simulink model "fft_wideband_real"  (R2012b)
settings: Solver=ode45  StartTime=0.0  StopTime=19999  RelTol=1e-3
undefined symbols (not defined in the file): fft_wideband_real_shift_schedule_user_data_out
libraries: xbsIndex_r4 x8703, xbsReplacements_r4 x36, xps_library x24, dspsigops x16, simulink_xsg_bridge x1
(part 2 of 51)

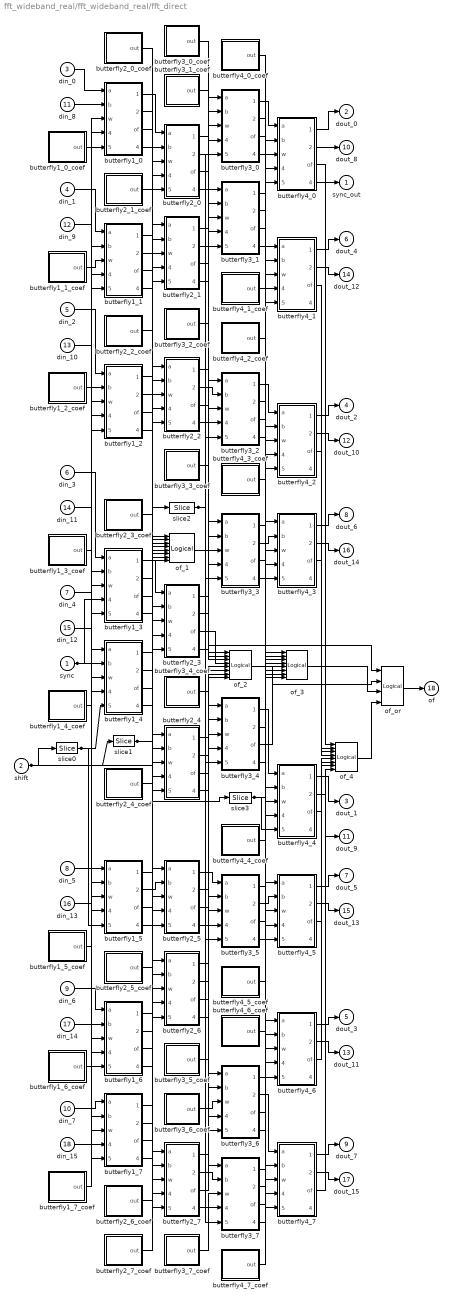
== system fft_wideband_real/fft_wideband_real/fft_direct ==
  sync : Inport
  shift : Inport  Port=2
  din_0 : Inport  Port=3
  din_1 : Inport  Port=4
  din_2 : Inport  Port=5
  din_3 : Inport  Port=6
  din_4 : Inport  Port=7
  din_5 : Inport  Port=8
  din_6 : Inport  Port=9
  din_7 : Inport  Port=10
  din_8 : Inport  Port=11
  din_9 : Inport  Port=12
  din_10 : Inport  Port=13
  din_11 : Inport  Port=14
  din_12 : Inport  Port=15
  din_13 : Inport  Port=16
  din_14 : Inport  Port=17
  din_15 : Inport  Port=18
  butterfly1_0 : Subsystem
      settings: AttributesFormatString=|
      | twiddle_pass_through
      | coeffs in slices
      | Bit growth:0
  butterfly1_0_coef : Subsystem
  butterfly1_1 : Subsystem
      settings: AttributesFormatString=|
      | twiddle_pass_through
      | coeffs in slices
      | Bit growth:0
  butterfly1_1_coef : Subsystem
  butterfly1_2 : Subsystem
      settings: AttributesFormatString=|
      | twiddle_pass_through
      | coeffs in slices
      | Bit growth:0
  butterfly1_2_coef : Subsystem
  butterfly1_3 : Subsystem
      settings: AttributesFormatString=|
      | twiddle_pass_through
      | coeffs in slices
      | Bit growth:0
  butterfly1_3_coef : Subsystem
  butterfly1_4 : Subsystem
      settings: AttributesFormatString=|
      | twiddle_pass_through
      | coeffs in slices
      | Bit growth:0
  butterfly1_4_coef : Subsystem
  butterfly1_5 : Subsystem
      settings: AttributesFormatString=|
      | twiddle_pass_through
      | coeffs in slices
      | Bit growth:0
  butterfly1_5_coef : Subsystem
  butterfly1_6 : Subsystem
      settings: AttributesFormatString=|
      | twiddle_pass_through
      | coeffs in slices
      | Bit growth:0
  butterfly1_6_coef : Subsystem
  butterfly1_7 : Subsystem
      settings: AttributesFormatString=|
      | twiddle_pass_through
      | coeffs in slices
      | Bit growth:0
  butterfly1_7_coef : Subsystem
  butterfly2_0 : Subsystem
      settings: AttributesFormatString=|
      | twiddle_pass_through
      | coeffs in slices
      | Bit growth:0
  butterfly2_0_coef : Subsystem
  butterfly2_1 : Subsystem
      settings: AttributesFormatString=|
      | twiddle_pass_through
      | coeffs in slices
      | Bit growth:0
  butterfly2_1_coef : Subsystem
  butterfly2_2 : Subsystem
      settings: AttributesFormatString=|
      | twiddle_pass_through
      | coeffs in slices
      | Bit growth:0
  butterfly2_2_coef : Subsystem
  butterfly2_3 : Subsystem
      settings: AttributesFormatString=|
      | twiddle_pass_through
      | coeffs in slices
      | Bit growth:0
  butterfly2_3_coef : Subsystem
  butterfly2_4 : Subsystem
      settings: AttributesFormatString=|
      | twiddle_coeff_1
      | coeffs in slices
      | Bit growth:0
  butterfly2_4_coef : Subsystem
  butterfly2_5 : Subsystem
      settings: AttributesFormatString=|
      | twiddle_coeff_1
      | coeffs in slices
      | Bit growth:0
  butterfly2_5_coef : Subsystem
  butterfly2_6 : Subsystem
      settings: AttributesFormatString=|
      | twiddle_coeff_1
      | coeffs in slices
      | Bit growth:0
  butterfly2_6_coef : Subsystem
  butterfly2_7 : Subsystem
      settings: AttributesFormatString=|
      | twiddle_coeff_1
      | coeffs in slices
      | Bit growth:0
  butterfly2_7_coef : Subsystem
  butterfly3_0 : Subsystem
      settings: AttributesFormatString=|
      | twiddle_general_4mult
      | coeffs in slices
      | Bit growth:0
  butterfly3_0_coef : Subsystem
  butterfly3_1 : Subsystem
      settings: AttributesFormatString=|
      | twiddle_general_4mult
      | coeffs in slices
      | Bit growth:0
  butterfly3_1_coef : Subsystem
  butterfly3_2 : Subsystem
      settings: AttributesFormatString=|
      | twiddle_general_4mult
      | coeffs in slices
      | Bit growth:0
  butterfly3_2_coef : Subsystem
  butterfly3_3 : Subsystem
      settings: AttributesFormatString=|
      | twiddle_general_4mult
      | coeffs in slices
      | Bit growth:0
  butterfly3_3_coef : Subsystem
  butterfly3_4 : Subsystem
      settings: AttributesFormatString=|
      | twiddle_general_4mult
      | coeffs in slices
      | Bit growth:0
  butterfly3_4_coef : Subsystem
  butterfly3_5 : Subsystem
      settings: AttributesFormatString=|
      | twiddle_general_4mult
      | coeffs in slices
      | Bit growth:0
  butterfly3_5_coef : Subsystem
  butterfly3_6 : Subsystem
      settings: AttributesFormatString=|
      | twiddle_general_4mult
      | coeffs in slices
      | Bit growth:0
  butterfly3_6_coef : Subsystem
  butterfly3_7 : Subsystem
      settings: AttributesFormatString=|
      | twiddle_general_4mult
      | coeffs in slices
      | Bit growth:0
  butterfly3_7_coef : Subsystem
  butterfly4_0 : Subsystem
      settings: AttributesFormatString=|
      | twiddle_general_4mult
      | coeffs in slices
      | Bit growth:0
  butterfly4_0_coef : Subsystem
  butterfly4_1 : Subsystem
      settings: AttributesFormatString=|
      | twiddle_general_4mult
      | coeffs in slices
      | Bit growth:0
  butterfly4_1_coef : Subsystem
  butterfly4_2 : Subsystem
      settings: AttributesFormatString=|
      | twiddle_general_4mult
      | coeffs in slices
      | Bit growth:0
  butterfly4_2_coef : Subsystem
  butterfly4_3 : Subsystem
      settings: AttributesFormatString=|
      | twiddle_general_4mult
      | coeffs in slices
      | Bit growth:0
  butterfly4_3_coef : Subsystem
  butterfly4_4 : Subsystem
      settings: AttributesFormatString=|
      | twiddle_general_4mult
      | coeffs in slices
      | Bit growth:0
  butterfly4_4_coef : Subsystem
  butterfly4_5 : Subsystem
      settings: AttributesFormatString=|
      | twiddle_general_4mult
      | coeffs in slices
      | Bit growth:0
  butterfly4_5_coef : Subsystem
  butterfly4_6 : Subsystem
      settings: AttributesFormatString=|
      | twiddle_general_4mult
      | coeffs in slices
      | Bit growth:0
  butterfly4_6_coef : Subsystem
  butterfly4_7 : Subsystem
      settings: AttributesFormatString=|
      | twiddle_general_4mult
      | coeffs in slices
      | Bit growth:0
  butterfly4_7_coef : Subsystem
  of_{1..4} (4 alike) : xbsIndex_r4/Logical  logical_function=OR  inputs=8  en=off  latency=1  precision=Full  arith_type=Unsigned  n_bits=16  bin_pt=0  align_bp=on  dbl_ovrd=off  block_type=logical
  of_or : xbsIndex_r4/Logical  logical_function=OR  inputs=4  en=off  latency=0  precision=Full  arith_type=Unsigned  n_bits=16  bin_pt=0  align_bp=on  dbl_ovrd=off  block_type=logical
  slice0 : xbsIndex_r4/Slice  nbits=1  boolean_output=on  mode=Lower Bit Location + Width  bit1=0  base1=MSB of Input  bit0=0  base0=LSB of Input  dbl_ovrd=off  block_type=slice
  slice1 : xbsIndex_r4/Slice  nbits=1  boolean_output=on  mode=Lower Bit Location + Width  bit1=0  base1=MSB of Input  bit0=1  base0=LSB of Input  dbl_ovrd=off  block_type=slice
  slice2 : xbsIndex_r4/Slice  nbits=1  boolean_output=on  mode=Lower Bit Location + Width  bit1=0  base1=MSB of Input  bit0=2  base0=LSB of Input  dbl_ovrd=off  block_type=slice
  slice3 : xbsIndex_r4/Slice  nbits=1  boolean_output=on  mode=Lower Bit Location + Width  bit1=0  base1=MSB of Input  bit0=3  base0=LSB of Input  dbl_ovrd=off  block_type=slice
  sync_out : Outport
  dout_0 : Outport  Port=2
  dout_1 : Outport  Port=3
  dout_2 : Outport  Port=4
  dout_3 : Outport  Port=5
  dout_4 : Outport  Port=6
  dout_5 : Outport  Port=7
  dout_6 : Outport  Port=8
  dout_7 : Outport  Port=9
  dout_8 : Outport  Port=10
  dout_9 : Outport  Port=11
  dout_10 : Outport  Port=12
  dout_11 : Outport  Port=13
  dout_12 : Outport  Port=14
  dout_13 : Outport  Port=15
  dout_14 : Outport  Port=16
  dout_15 : Outport  Port=17
  of : Outport  Port=18
  wires:
  din_0/1 -> butterfly1_0/1(a)
  din_8/1 -> butterfly1_0/2(b)
  butterfly1_0_coef/1(out) -> butterfly1_0/3(w)
  din_1/1 -> butterfly1_1/1(a)
  din_9/1 -> butterfly1_1/2(b)
  butterfly1_1_coef/1(out) -> butterfly1_1/3(w)
  din_2/1 -> butterfly1_2/1(a)
  din_10/1 -> butterfly1_2/2(b)
  butterfly1_2_coef/1(out) -> butterfly1_2/3(w)
  din_3/1 -> butterfly1_3/1(a)
  din_11/1 -> butterfly1_3/2(b)
  butterfly1_3_coef/1(out) -> butterfly1_3/3(w)
  din_4/1 -> butterfly1_4/1(a)
  din_12/1 -> butterfly1_4/2(b)
  butterfly1_4_coef/1(out) -> butterfly1_4/3(w)
  din_5/1 -> butterfly1_5/1(a)
  din_13/1 -> butterfly1_5/2(b)
  butterfly1_5_coef/1(out) -> butterfly1_5/3(w)
  din_6/1 -> butterfly1_6/1(a)
  din_14/1 -> butterfly1_6/2(b)
  butterfly1_6_coef/1(out) -> butterfly1_6/3(w)
  din_7/1 -> butterfly1_7/1(a)
  din_15/1 -> butterfly1_7/2(b)
  butterfly1_7_coef/1(out) -> butterfly1_7/3(w)
  butterfly1_0/3(of) -> of_1/1
  butterfly1_1/3(of) -> of_1/2
  butterfly1_2/3(of) -> of_1/3
  butterfly1_3/3(of) -> of_1/4
  butterfly1_4/3(of) -> of_1/5
  butterfly1_5/3(of) -> of_1/6
  butterfly1_6/3(of) -> of_1/7
  butterfly1_7/3(of) -> of_1/8
  butterfly1_0/1(a+bw) -> butterfly2_0/1(a)
  butterfly1_4/1(a+bw) -> butterfly2_0/2(b)
  butterfly2_0_coef/1(out) -> butterfly2_0/3(w)
  butterfly1_0/4(sync_out) -> butterfly2_0/4(sync)
  butterfly1_1/1(a+bw) -> butterfly2_1/1(a)
  butterfly1_5/1(a+bw) -> butterfly2_1/2(b)
  butterfly2_1_coef/1(out) -> butterfly2_1/3(w)
  butterfly1_1/4(sync_out) -> butterfly2_1/4(sync)
  butterfly1_2/1(a+bw) -> butterfly2_2/1(a)
  butterfly1_6/1(a+bw) -> butterfly2_2/2(b)
  butterfly2_2_coef/1(out) -> butterfly2_2/3(w)
  butterfly1_2/4(sync_out) -> butterfly2_2/4(sync)
  butterfly1_3/1(a+bw) -> butterfly2_3/1(a)
  butterfly1_7/1(a+bw) -> butterfly2_3/2(b)
  butterfly2_3_coef/1(out) -> butterfly2_3/3(w)
  butterfly1_3/4(sync_out) -> butterfly2_3/4(sync)
  butterfly1_0/2(a-bw) -> butterfly2_4/1(a)
  butterfly1_4/2(a-bw) -> butterfly2_4/2(b)
  butterfly2_4_coef/1(out) -> butterfly2_4/3(w)
  butterfly1_4/4(sync_out) -> butterfly2_4/4(sync)
  butterfly1_1/2(a-bw) -> butterfly2_5/1(a)
  butterfly1_5/2(a-bw) -> butterfly2_5/2(b)
  butterfly2_5_coef/1(out) -> butterfly2_5/3(w)
  butterfly1_5/4(sync_out) -> butterfly2_5/4(sync)
  butterfly1_2/2(a-bw) -> butterfly2_6/1(a)
  butterfly1_6/2(a-bw) -> butterfly2_6/2(b)
  butterfly2_6_coef/1(out) -> butterfly2_6/3(w)
  butterfly1_6/4(sync_out) -> butterfly2_6/4(sync)
  butterfly1_3/2(a-bw) -> butterfly2_7/1(a)
  butterfly1_7/2(a-bw) -> butterfly2_7/2(b)
  butterfly2_7_coef/1(out) -> butterfly2_7/3(w)
  butterfly1_7/4(sync_out) -> butterfly2_7/4(sync)
  butterfly2_0/3(of) -> of_2/1
  butterfly2_1/3(of) -> of_2/2
  butterfly2_2/3(of) -> of_2/3
  butterfly2_3/3(of) -> of_2/4
  butterfly2_4/3(of) -> of_2/5
  butterfly2_5/3(of) -> of_2/6
  butterfly2_6/3(of) -> of_2/7
  butterfly2_7/3(of) -> of_2/8
  butterfly2_0/1(a+bw) -> butterfly3_0/1(a)
  butterfly2_2/1(a+bw) -> butterfly3_0/2(b)
  butterfly3_0_coef/1(out) -> butterfly3_0/3(w)
  butterfly2_0/4(sync_out) -> butterfly3_0/4(sync)
  butterfly2_1/1(a+bw) -> butterfly3_1/1(a)
  butterfly2_3/1(a+bw) -> butterfly3_1/2(b)
  butterfly3_1_coef/1(out) -> butterfly3_1/3(w)
  butterfly2_1/4(sync_out) -> butterfly3_1/4(sync)
  butterfly2_0/2(a-bw) -> butterfly3_2/1(a)
  butterfly2_2/2(a-bw) -> butterfly3_2/2(b)
  butterfly3_2_coef/1(out) -> butterfly3_2/3(w)
  butterfly2_2/4(sync_out) -> butterfly3_2/4(sync)
  butterfly2_1/2(a-bw) -> butterfly3_3/1(a)
  butterfly2_3/2(a-bw) -> butterfly3_3/2(b)
  butterfly3_3_coef/1(out) -> butterfly3_3/3(w)
  butterfly2_3/4(sync_out) -> butterfly3_3/4(sync)
  butterfly2_4/1(a+bw) -> butterfly3_4/1(a)
  butterfly2_6/1(a+bw) -> butterfly3_4/2(b)
  butterfly3_4_coef/1(out) -> butterfly3_4/3(w)
  butterfly2_4/4(sync_out) -> butterfly3_4/4(sync)
  butterfly2_5/1(a+bw) -> butterfly3_5/1(a)
  butterfly2_7/1(a+bw) -> butterfly3_5/2(b)
  butterfly3_5_coef/1(out) -> butterfly3_5/3(w)
  butterfly2_5/4(sync_out) -> butterfly3_5/4(sync)
  butterfly2_4/2(a-bw) -> butterfly3_6/1(a)
  butterfly2_6/2(a-bw) -> butterfly3_6/2(b)
  butterfly3_6_coef/1(out) -> butterfly3_6/3(w)
  butterfly2_6/4(sync_out) -> butterfly3_6/4(sync)
  butterfly2_5/2(a-bw) -> butterfly3_7/1(a)
  butterfly2_7/2(a-bw) -> butterfly3_7/2(b)
  butterfly3_7_coef/1(out) -> butterfly3_7/3(w)
  butterfly2_7/4(sync_out) -> butterfly3_7/4(sync)
  butterfly3_0/3(of) -> of_3/1
  butterfly3_1/3(of) -> of_3/2
  butterfly3_2/3(of) -> of_3/3
  butterfly3_3/3(of) -> of_3/4
  butterfly3_4/3(of) -> of_3/5
  butterfly3_5/3(of) -> of_3/6
  butterfly3_6/3(of) -> of_3/7
  butterfly3_7/3(of) -> of_3/8
  butterfly3_0/1(a+bw) -> butterfly4_0/1(a)
  butterfly3_1/1(a+bw) -> butterfly4_0/2(b)
  butterfly4_0_coef/1(out) -> butterfly4_0/3(w)
  butterfly3_0/4(sync_out) -> butterfly4_0/4(sync)
  butterfly4_0/4(sync_out) -> sync_out/1
  butterfly3_0/2(a-bw) -> butterfly4_1/1(a)
  butterfly3_1/2(a-bw) -> butterfly4_1/2(b)
  butterfly4_1_coef/1(out) -> butterfly4_1/3(w)
  butterfly3_1/4(sync_out) -> butterfly4_1/4(sync)
  butterfly3_2/1(a+bw) -> butterfly4_2/1(a)
  butterfly3_3/1(a+bw) -> butterfly4_2/2(b)
  butterfly4_2_coef/1(out) -> butterfly4_2/3(w)
  butterfly3_2/4(sync_out) -> butterfly4_2/4(sync)
  butterfly3_2/2(a-bw) -> butterfly4_3/1(a)
  butterfly3_3/2(a-bw) -> butterfly4_3/2(b)
  butterfly4_3_coef/1(out) -> butterfly4_3/3(w)
  butterfly3_3/4(sync_out) -> butterfly4_3/4(sync)
  butterfly3_4/1(a+bw) -> butterfly4_4/1(a)
  butterfly3_5/1(a+bw) -> butterfly4_4/2(b)
  butterfly4_4_coef/1(out) -> butterfly4_4/3(w)
  butterfly3_4/4(sync_out) -> butterfly4_4/4(sync)
  butterfly3_4/2(a-bw) -> butterfly4_5/1(a)
  butterfly3_5/2(a-bw) -> butterfly4_5/2(b)
  butterfly4_5_coef/1(out) -> butterfly4_5/3(w)
  butterfly3_5/4(sync_out) -> butterfly4_5/4(sync)
  butterfly3_6/1(a+bw) -> butterfly4_6/1(a)
  butterfly3_7/1(a+bw) -> butterfly4_6/2(b)
  butterfly4_6_coef/1(out) -> butterfly4_6/3(w)
  butterfly3_6/4(sync_out) -> butterfly4_6/4(sync)
  butterfly3_6/2(a-bw) -> butterfly4_7/1(a)
  butterfly3_7/2(a-bw) -> butterfly4_7/2(b)
  butterfly4_7_coef/1(out) -> butterfly4_7/3(w)
  butterfly3_7/4(sync_out) -> butterfly4_7/4(sync)
  butterfly4_0/3(of) -> of_4/1
  butterfly4_1/3(of) -> of_4/2
  butterfly4_2/3(of) -> of_4/3
  butterfly4_3/3(of) -> of_4/4
  butterfly4_4/3(of) -> of_4/5
  butterfly4_5/3(of) -> of_4/6
  butterfly4_6/3(of) -> of_4/7
  butterfly4_7/3(of) -> of_4/8
  of_1/1 -> of_or/1
  of_2/1 -> of_or/2
  of_3/1 -> of_or/3
  of_4/1 -> of_or/4
  of_or/1 -> of/1
  butterfly4_0/1(a+bw) -> dout_0/1
  butterfly4_4/1(a+bw) -> dout_1/1
  butterfly4_2/1(a+bw) -> dout_2/1
  butterfly4_6/1(a+bw) -> dout_3/1
  butterfly4_1/1(a+bw) -> dout_4/1
  butterfly4_5/1(a+bw) -> dout_5/1
  butterfly4_3/1(a+bw) -> dout_6/1
  butterfly4_7/1(a+bw) -> dout_7/1
  butterfly4_0/2(a-bw) -> dout_8/1
  butterfly4_4/2(a-bw) -> dout_9/1
  butterfly4_2/2(a-bw) -> dout_10/1
  butterfly4_6/2(a-bw) -> dout_11/1
  butterfly4_1/2(a-bw) -> dout_12/1
  butterfly4_5/2(a-bw) -> dout_13/1
  butterfly4_3/2(a-bw) -> dout_14/1
  butterfly4_7/2(a-bw) -> dout_15/1
  slice3/1 -> butterfly4_0/5(shift), butterfly4_1/5(shift), butterfly4_2/5(shift), butterfly4_3/5(shift), butterfly4_4/5(shift), butterfly4_5/5(shift), butterfly4_6/5(shift), butterfly4_7/5(shift)
  slice2/1 -> butterfly3_0/5(shift), butterfly3_1/5(shift), butterfly3_2/5(shift), butterfly3_3/5(shift), butterfly3_4/5(shift), butterfly3_5/5(shift), butterfly3_6/5(shift), butterfly3_7/5(shift)
  slice1/1 -> butterfly2_0/5(shift), butterfly2_1/5(shift), butterfly2_2/5(shift), butterfly2_3/5(shift), butterfly2_4/5(shift), butterfly2_5/5(shift), butterfly2_6/5(shift), butterfly2_7/5(shift)
  slice0/1 -> butterfly1_0/5(shift), butterfly1_1/5(shift), butterfly1_2/5(shift), butterfly1_3/5(shift), butterfly1_4/5(shift), butterfly1_5/5(shift), butterfly1_6/5(shift), butterfly1_7/5(shift)
  sync/1 -> butterfly1_0/4(sync), butterfly1_1/4(sync), butterfly1_2/4(sync), butterfly1_3/4(sync), butterfly1_4/4(sync), butterfly1_5/4(sync), butterfly1_6/4(sync), butterfly1_7/4(sync)
  shift/1 -> slice0/1, slice1/1, slice2/1, slice3/1

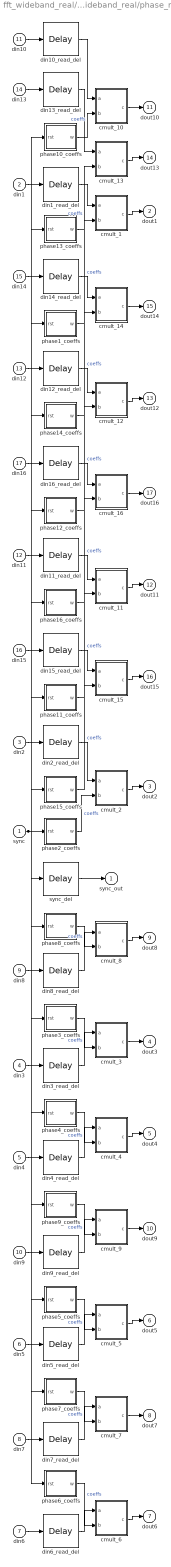
== system fft_wideband_real/fft_wideband_real/phase_mult ==
  sync : Inport
  din1 : Inport  Port=2
  din2 : Inport  Port=3
  din3 : Inport  Port=4
  din4 : Inport  Port=5
  din5 : Inport  Port=6
  din6 : Inport  Port=7
  din7 : Inport  Port=8
  din8 : Inport  Port=9
  din9 : Inport  Port=10
  din10 : Inport  Port=11
  din11 : Inport  Port=12
  din12 : Inport  Port=13
  din13 : Inport  Port=14
  din14 : Inport  Port=15
  din15 : Inport  Port=16
  din16 : Inport  Port=17
  cmult_1 : Subsystem
  cmult_10 : Subsystem
  cmult_11 : Subsystem
  cmult_12 : Subsystem
  cmult_13 : Subsystem
  cmult_14 : Subsystem
  cmult_15 : Subsystem
  cmult_16 : Subsystem
  cmult_2 : Subsystem
  cmult_3 : Subsystem
  cmult_4 : Subsystem
  cmult_5 : Subsystem
  cmult_6 : Subsystem
  cmult_7 : Subsystem
  cmult_8 : Subsystem
  cmult_9 : Subsystem
  din10_read_del : xbsIndex_r4/Delay  rst=off  infoeditControl=Selection of Reset will increase slice count due to use of real FFs and instead of SRLs  en=off  latency=2  dbl_ovrd=off  reg_retiming=off  block_type=delay
  din11_read_del : xbsIndex_r4/Delay  rst=off  infoeditControl=Selection of Reset will increase slice count due to use of real FFs and instead of SRLs  en=off  latency=2  dbl_ovrd=off  reg_retiming=off  block_type=delay
  din12_read_del : xbsIndex_r4/Delay  rst=off  infoeditControl=Selection of Reset will increase slice count due to use of real FFs and instead of SRLs  en=off  latency=2  dbl_ovrd=off  reg_retiming=off  block_type=delay
  din13_read_del : xbsIndex_r4/Delay  rst=off  infoeditControl=Selection of Reset will increase slice count due to use of real FFs and instead of SRLs  en=off  latency=2  dbl_ovrd=off  reg_retiming=off  block_type=delay
  din14_read_del : xbsIndex_r4/Delay  rst=off  infoeditControl=Selection of Reset will increase slice count due to use of real FFs and instead of SRLs  en=off  latency=2  dbl_ovrd=off  reg_retiming=off  block_type=delay
  din15_read_del : xbsIndex_r4/Delay  rst=off  infoeditControl=Selection of Reset will increase slice count due to use of real FFs and instead of SRLs  en=off  latency=2  dbl_ovrd=off  reg_retiming=off  block_type=delay
  din16_read_del : xbsIndex_r4/Delay  rst=off  infoeditControl=Selection of Reset will increase slice count due to use of real FFs and instead of SRLs  en=off  latency=2  dbl_ovrd=off  reg_retiming=off  block_type=delay
  din1_read_del : xbsIndex_r4/Delay  rst=off  infoeditControl=Selection of Reset will increase slice count due to use of real FFs and instead of SRLs  en=off  latency=2  dbl_ovrd=off  reg_retiming=off  block_type=delay
  din2_read_del : xbsIndex_r4/Delay  rst=off  infoeditControl=Selection of Reset will increase slice count due to use of real FFs and instead of SRLs  en=off  latency=2  dbl_ovrd=off  reg_retiming=off  block_type=delay
  din3_read_del : xbsIndex_r4/Delay  rst=off  infoeditControl=Selection of Reset will increase slice count due to use of real FFs and instead of SRLs  en=off  latency=2  dbl_ovrd=off  reg_retiming=off  block_type=delay
  din4_read_del : xbsIndex_r4/Delay  rst=off  infoeditControl=Selection of Reset will increase slice count due to use of real FFs and instead of SRLs  en=off  latency=2  dbl_ovrd=off  reg_retiming=off  block_type=delay
  din5_read_del : xbsIndex_r4/Delay  rst=off  infoeditControl=Selection of Reset will increase slice count due to use of real FFs and instead of SRLs  en=off  latency=2  dbl_ovrd=off  reg_retiming=off  block_type=delay
  din6_read_del : xbsIndex_r4/Delay  rst=off  infoeditControl=Selection of Reset will increase slice count due to use of real FFs and instead of SRLs  en=off  latency=2  dbl_ovrd=off  reg_retiming=off  block_type=delay
  din7_read_del : xbsIndex_r4/Delay  rst=off  infoeditControl=Selection of Reset will increase slice count due to use of real FFs and instead of SRLs  en=off  latency=2  dbl_ovrd=off  reg_retiming=off  block_type=delay
  din8_read_del : xbsIndex_r4/Delay  rst=off  infoeditControl=Selection of Reset will increase slice count due to use of real FFs and instead of SRLs  en=off  latency=2  dbl_ovrd=off  reg_retiming=off  block_type=delay
  din9_read_del : xbsIndex_r4/Delay  rst=off  infoeditControl=Selection of Reset will increase slice count due to use of real FFs and instead of SRLs  en=off  latency=2  dbl_ovrd=off  reg_retiming=off  block_type=delay
  phase10_coeffs : Subsystem
      settings: AttributesFormatString=64 @ (18,17)
  phase11_coeffs : Subsystem
      settings: AttributesFormatString=64 @ (18,17)
  phase12_coeffs : Subsystem
      settings: AttributesFormatString=64 @ (18,17)
  phase13_coeffs : Subsystem
      settings: AttributesFormatString=64 @ (18,17)
  phase14_coeffs : Subsystem
      settings: AttributesFormatString=64 @ (18,17)
  phase15_coeffs : Subsystem
      settings: AttributesFormatString=64 @ (18,17)
  phase16_coeffs : Subsystem
      settings: AttributesFormatString=64 @ (18,17)
  phase1_coeffs : Subsystem
      settings: AttributesFormatString=64 @ (18,17)
  phase2_coeffs : Subsystem
      settings: AttributesFormatString=64 @ (18,17)
  phase3_coeffs : Subsystem
      settings: AttributesFormatString=64 @ (18,17)
  phase4_coeffs : Subsystem
      settings: AttributesFormatString=64 @ (18,17)
  phase5_coeffs : Subsystem
      settings: AttributesFormatString=64 @ (18,17)
  phase6_coeffs : Subsystem
      settings: AttributesFormatString=64 @ (18,17)
  phase7_coeffs : Subsystem
      settings: AttributesFormatString=64 @ (18,17)
  phase8_coeffs : Subsystem
      settings: AttributesFormatString=64 @ (18,17)
  phase9_coeffs : Subsystem
      settings: AttributesFormatString=64 @ (18,17)
  sync_del : xbsIndex_r4/Delay  rst=off  infoeditControl=Selection of Reset will increase slice count due to use of real FFs and instead of SRLs  en=off  latency=8  dbl_ovrd=off  reg_retiming=off  block_type=delay
  sync_out : Outport
  dout1 : Outport  Port=2
  dout2 : Outport  Port=3
  dout3 : Outport  Port=4
  dout4 : Outport  Port=5
  dout5 : Outport  Port=6
  dout6 : Outport  Port=7
  dout7 : Outport  Port=8
  dout8 : Outport  Port=9
  dout9 : Outport  Port=10
  dout10 : Outport  Port=11
  dout11 : Outport  Port=12
  dout12 : Outport  Port=13
  dout13 : Outport  Port=14
  dout14 : Outport  Port=15
  dout15 : Outport  Port=16
  dout16 : Outport  Port=17
  wires:
  sync/1 -> sync_del/1, phase16_coeffs/1(rst), phase15_coeffs/1(rst), phase14_coeffs/1(rst), phase13_coeffs/1(rst), phase12_coeffs/1(rst), phase11_coeffs/1(rst), phase10_coeffs/1(rst), phase9_coeffs/1(rst), phase8_coeffs/1(rst), phase7_coeffs/1(rst), phase6_coeffs/1(rst), phase5_coeffs/1(rst), phase4_coeffs/1(rst), phase3_coeffs/1(rst), phase2_coeffs/1(rst), phase1_coeffs/1(rst)
  sync_del/1 -> sync_out/1
  cmult_16/1(c) -> dout16/1
  phase16_coeffs/1(w) -> cmult_16/2(b)  "coeffs"
  din16_read_del/1 -> cmult_16/1(a)
  din16/1 -> din16_read_del/1
  cmult_15/1(c) -> dout15/1
  phase15_coeffs/1(w) -> cmult_15/2(b)  "coeffs"
  din15_read_del/1 -> cmult_15/1(a)
  din15/1 -> din15_read_del/1
  cmult_14/1(c) -> dout14/1
  phase14_coeffs/1(w) -> cmult_14/2(b)  "coeffs"
  din14_read_del/1 -> cmult_14/1(a)
  din14/1 -> din14_read_del/1
  cmult_13/1(c) -> dout13/1
  phase13_coeffs/1(w) -> cmult_13/2(b)  "coeffs"
  din13_read_del/1 -> cmult_13/1(a)
  din13/1 -> din13_read_del/1
  cmult_12/1(c) -> dout12/1
  phase12_coeffs/1(w) -> cmult_12/2(b)  "coeffs"
  din12_read_del/1 -> cmult_12/1(a)
  din12/1 -> din12_read_del/1
  cmult_11/1(c) -> dout11/1
  phase11_coeffs/1(w) -> cmult_11/2(b)  "coeffs"
  din11_read_del/1 -> cmult_11/1(a)
  din11/1 -> din11_read_del/1
  cmult_10/1(c) -> dout10/1
  phase10_coeffs/1(w) -> cmult_10/2(b)  "coeffs"
  din10_read_del/1 -> cmult_10/1(a)
  din10/1 -> din10_read_del/1
  cmult_9/1(c) -> dout9/1
  phase9_coeffs/1(w) -> cmult_9/2(b)  "coeffs"
  din9_read_del/1 -> cmult_9/1(a)
  din9/1 -> din9_read_del/1
  cmult_8/1(c) -> dout8/1
  phase8_coeffs/1(w) -> cmult_8/2(b)  "coeffs"
  din8_read_del/1 -> cmult_8/1(a)
  din8/1 -> din8_read_del/1
  cmult_7/1(c) -> dout7/1
  phase7_coeffs/1(w) -> cmult_7/2(b)  "coeffs"
  din7_read_del/1 -> cmult_7/1(a)
  din7/1 -> din7_read_del/1
  cmult_6/1(c) -> dout6/1
  phase6_coeffs/1(w) -> cmult_6/2(b)  "coeffs"
  din6_read_del/1 -> cmult_6/1(a)
  din6/1 -> din6_read_del/1
  cmult_5/1(c) -> dout5/1
  phase5_coeffs/1(w) -> cmult_5/2(b)  "coeffs"
  din5_read_del/1 -> cmult_5/1(a)
  din5/1 -> din5_read_del/1
  cmult_4/1(c) -> dout4/1
  phase4_coeffs/1(w) -> cmult_4/2(b)  "coeffs"
  din4_read_del/1 -> cmult_4/1(a)
  din4/1 -> din4_read_del/1
  cmult_3/1(c) -> dout3/1
  phase3_coeffs/1(w) -> cmult_3/2(b)  "coeffs"
  din3_read_del/1 -> cmult_3/1(a)
  din3/1 -> din3_read_del/1
  cmult_2/1(c) -> dout2/1
  phase2_coeffs/1(w) -> cmult_2/2(b)  "coeffs"
  din2_read_del/1 -> cmult_2/1(a)
  din2/1 -> din2_read_del/1
  cmult_1/1(c) -> dout1/1
  phase1_coeffs/1(w) -> cmult_1/2(b)  "coeffs"
  din1_read_del/1 -> cmult_1/1(a)
  din1/1 -> din1_read_del/1

== system fft_wideband_real/fft_wideband_real/to_workspace_complex16 ==
  biplex_out2 : Inport
  c_to_ri : Subsystem
  imag_gateway : xbsIndex_r4/Gateway Out  inherit_from_input=on  hdl_port=off  timing_constraint=None  locs_specified=off  LOCs={}  UseAsDAC=off  DACChannel='1'  block_type=gatewayout
  real_gateway : xbsIndex_r4/Gateway Out  inherit_from_input=on  hdl_port=off  timing_constraint=None  locs_specified=off  LOCs={}  UseAsDAC=off  DACChannel='1'  block_type=gatewayout
  ri_to_c : RealImagToComplex
  workspace_output : ToWorkspace  VariableName=biplex_out2  SampleTime=-1
  _o : Outport
  wires:
  biplex_out2/1 -> c_to_ri/1(c), _o/1
  ri_to_c/1 -> workspace_output/1  "cplx"
  imag_gateway/1 -> ri_to_c/2
  real_gateway/1 -> ri_to_c/1
  c_to_ri/2(im) -> imag_gateway/1  "c_to_ri_out2"
  c_to_ri/1(re) -> real_gateway/1  "c_to_ri_out1"

== system fft_wideband_real/fft_wideband_real/to_workspace_complex17 ==
  biplex_out1 : Inport
  c_to_ri : Subsystem
  imag_gateway : xbsIndex_r4/Gateway Out  inherit_from_input=on  hdl_port=off  timing_constraint=None  locs_specified=off  LOCs={}  UseAsDAC=off  DACChannel='1'  block_type=gatewayout
  real_gateway : xbsIndex_r4/Gateway Out  inherit_from_input=on  hdl_port=off  timing_constraint=None  locs_specified=off  LOCs={}  UseAsDAC=off  DACChannel='1'  block_type=gatewayout
  ri_to_c : RealImagToComplex
  workspace_output : ToWorkspace  VariableName=biplex_out1  SampleTime=-1
  _o : Outport
  wires:
  biplex_out1/1 -> c_to_ri/1(c), _o/1
  ri_to_c/1 -> workspace_output/1  "cplx"
  imag_gateway/1 -> ri_to_c/2
  real_gateway/1 -> ri_to_c/1
  c_to_ri/2(im) -> imag_gateway/1  "c_to_ri_out2"
  c_to_ri/1(re) -> real_gateway/1  "c_to_ri_out1"

== system fft_wideband_real/fft_wideband_real/to_workspace_complex18 ==
  biplex_out4 : Inport
  c_to_ri : Subsystem
  imag_gateway : xbsIndex_r4/Gateway Out  inherit_from_input=on  hdl_port=off  timing_constraint=None  locs_specified=off  LOCs={}  UseAsDAC=off  DACChannel='1'  block_type=gatewayout
  real_gateway : xbsIndex_r4/Gateway Out  inherit_from_input=on  hdl_port=off  timing_constraint=None  locs_specified=off  LOCs={}  UseAsDAC=off  DACChannel='1'  block_type=gatewayout
  ri_to_c : RealImagToComplex
  workspace_output : ToWorkspace  VariableName=biplex_out4  SampleTime=-1
  _o : Outport
  wires:
  biplex_out4/1 -> c_to_ri/1(c), _o/1
  ri_to_c/1 -> workspace_output/1  "cplx"
  imag_gateway/1 -> ri_to_c/2
  real_gateway/1 -> ri_to_c/1
  c_to_ri/2(im) -> imag_gateway/1  "c_to_ri_out2"
  c_to_ri/1(re) -> real_gateway/1  "c_to_ri_out1"

== system fft_wideband_real/fft_wideband_real/to_workspace_complex19 ==
  biplex_out3 : Inport
  c_to_ri : Subsystem
  imag_gateway : xbsIndex_r4/Gateway Out  inherit_from_input=on  hdl_port=off  timing_constraint=None  locs_specified=off  LOCs={}  UseAsDAC=off  DACChannel='1'  block_type=gatewayout
  real_gateway : xbsIndex_r4/Gateway Out  inherit_from_input=on  hdl_port=off  timing_constraint=None  locs_specified=off  LOCs={}  UseAsDAC=off  DACChannel='1'  block_type=gatewayout
  ri_to_c : RealImagToComplex
  workspace_output : ToWorkspace  VariableName=biplex_out3  SampleTime=-1
  _o : Outport
  wires:
  biplex_out3/1 -> c_to_ri/1(c), _o/1
  ri_to_c/1 -> workspace_output/1  "cplx"
  imag_gateway/1 -> ri_to_c/2
  real_gateway/1 -> ri_to_c/1
  c_to_ri/2(im) -> imag_gateway/1  "c_to_ri_out2"
  c_to_ri/1(re) -> real_gateway/1  "c_to_ri_out1"

== system fft_wideband_real/fft_wideband_real/to_workspace_real1 ==
  biplex_sync_out : Inport
  gateway : xbsIndex_r4/Gateway Out  inherit_from_input=on  hdl_port=off  timing_constraint=None  locs_specified=off  LOCs={}  UseAsDAC=off  DACChannel='1'  block_type=gatewayout
  workspace_input : ToWorkspace  VariableName=biplex_sync_out  SampleTime=-1
  _o : Outport
  wires:
  biplex_sync_out/1 -> gateway/1, _o/1
  gateway/1 -> workspace_input/1

== system fft_wideband_real/multi_to_workspace_complex/to_workspace_cplx_1 ==
  out1 : Inport
  c_to_ri : Subsystem
  imag_gateway : xbsIndex_r4/Gateway Out  inherit_from_input=on  hdl_port=off  timing_constraint=None  locs_specified=off  LOCs={}  UseAsDAC=off  DACChannel='1'  block_type=gatewayout
  real_gateway : xbsIndex_r4/Gateway Out  inherit_from_input=on  hdl_port=off  timing_constraint=None  locs_specified=off  LOCs={}  UseAsDAC=off  DACChannel='1'  block_type=gatewayout
  ri_to_c : RealImagToComplex
  workspace_output : ToWorkspace  VariableName=out1  SampleTime=-1
  _o : Outport
  wires:
  out1/1 -> c_to_ri/1(c), _o/1
  ri_to_c/1 -> workspace_output/1  "cplx"
  imag_gateway/1 -> ri_to_c/2
  real_gateway/1 -> ri_to_c/1
  c_to_ri/2(im) -> imag_gateway/1  "c_to_ri_out2"
  c_to_ri/1(re) -> real_gateway/1  "c_to_ri_out1"

== system fft_wideband_real/multi_to_workspace_complex/to_workspace_cplx_10 ==
  out10 : Inport
  c_to_ri : Subsystem
  imag_gateway : xbsIndex_r4/Gateway Out  inherit_from_input=on  hdl_port=off  timing_constraint=None  locs_specified=off  LOCs={}  UseAsDAC=off  DACChannel='1'  block_type=gatewayout
  real_gateway : xbsIndex_r4/Gateway Out  inherit_from_input=on  hdl_port=off  timing_constraint=None  locs_specified=off  LOCs={}  UseAsDAC=off  DACChannel='1'  block_type=gatewayout
  ri_to_c : RealImagToComplex
  workspace_output : ToWorkspace  VariableName=out10  SampleTime=-1
  _o : Outport
  wires:
  out10/1 -> c_to_ri/1(c), _o/1
  ri_to_c/1 -> workspace_output/1  "cplx"
  imag_gateway/1 -> ri_to_c/2
  real_gateway/1 -> ri_to_c/1
  c_to_ri/2(im) -> imag_gateway/1  "c_to_ri_out2"
  c_to_ri/1(re) -> real_gateway/1  "c_to_ri_out1"

== system fft_wideband_real/multi_to_workspace_complex/to_workspace_cplx_11 ==
  out11 : Inport
  c_to_ri : Subsystem
  imag_gateway : xbsIndex_r4/Gateway Out  inherit_from_input=on  hdl_port=off  timing_constraint=None  locs_specified=off  LOCs={}  UseAsDAC=off  DACChannel='1'  block_type=gatewayout
  real_gateway : xbsIndex_r4/Gateway Out  inherit_from_input=on  hdl_port=off  timing_constraint=None  locs_specified=off  LOCs={}  UseAsDAC=off  DACChannel='1'  block_type=gatewayout
  ri_to_c : RealImagToComplex
  workspace_output : ToWorkspace  VariableName=out11  SampleTime=-1
  _o : Outport
  wires:
  out11/1 -> c_to_ri/1(c), _o/1
  ri_to_c/1 -> workspace_output/1  "cplx"
  imag_gateway/1 -> ri_to_c/2
  real_gateway/1 -> ri_to_c/1
  c_to_ri/2(im) -> imag_gateway/1  "c_to_ri_out2"
  c_to_ri/1(re) -> real_gateway/1  "c_to_ri_out1"

== system fft_wideband_real/multi_to_workspace_complex/to_workspace_cplx_12 ==
  out12 : Inport
  c_to_ri : Subsystem
  imag_gateway : xbsIndex_r4/Gateway Out  inherit_from_input=on  hdl_port=off  timing_constraint=None  locs_specified=off  LOCs={}  UseAsDAC=off  DACChannel='1'  block_type=gatewayout
  real_gateway : xbsIndex_r4/Gateway Out  inherit_from_input=on  hdl_port=off  timing_constraint=None  locs_specified=off  LOCs={}  UseAsDAC=off  DACChannel='1'  block_type=gatewayout
  ri_to_c : RealImagToComplex
  workspace_output : ToWorkspace  VariableName=out12  SampleTime=-1
  _o : Outport
  wires:
  out12/1 -> c_to_ri/1(c), _o/1
  ri_to_c/1 -> workspace_output/1  "cplx"
  imag_gateway/1 -> ri_to_c/2
  real_gateway/1 -> ri_to_c/1
  c_to_ri/2(im) -> imag_gateway/1  "c_to_ri_out2"
  c_to_ri/1(re) -> real_gateway/1  "c_to_ri_out1"

== system fft_wideband_real/multi_to_workspace_complex/to_workspace_cplx_13 ==
  out13 : Inport
  c_to_ri : Subsystem
  imag_gateway : xbsIndex_r4/Gateway Out  inherit_from_input=on  hdl_port=off  timing_constraint=None  locs_specified=off  LOCs={}  UseAsDAC=off  DACChannel='1'  block_type=gatewayout
  real_gateway : xbsIndex_r4/Gateway Out  inherit_from_input=on  hdl_port=off  timing_constraint=None  locs_specified=off  LOCs={}  UseAsDAC=off  DACChannel='1'  block_type=gatewayout
  ri_to_c : RealImagToComplex
  workspace_output : ToWorkspace  VariableName=out13  SampleTime=-1
  _o : Outport
  wires:
  out13/1 -> c_to_ri/1(c), _o/1
  ri_to_c/1 -> workspace_output/1  "cplx"
  imag_gateway/1 -> ri_to_c/2
  real_gateway/1 -> ri_to_c/1
  c_to_ri/2(im) -> imag_gateway/1  "c_to_ri_out2"
  c_to_ri/1(re) -> real_gateway/1  "c_to_ri_out1"

== system fft_wideband_real/multi_to_workspace_complex/to_workspace_cplx_14 ==
  out14 : Inport
  c_to_ri : Subsystem
  imag_gateway : xbsIndex_r4/Gateway Out  inherit_from_input=on  hdl_port=off  timing_constraint=None  locs_specified=off  LOCs={}  UseAsDAC=off  DACChannel='1'  block_type=gatewayout
  real_gateway : xbsIndex_r4/Gateway Out  inherit_from_input=on  hdl_port=off  timing_constraint=None  locs_specified=off  LOCs={}  UseAsDAC=off  DACChannel='1'  block_type=gatewayout
  ri_to_c : RealImagToComplex
  workspace_output : ToWorkspace  VariableName=out14  SampleTime=-1
  _o : Outport
  wires:
  out14/1 -> c_to_ri/1(c), _o/1
  ri_to_c/1 -> workspace_output/1  "cplx"
  imag_gateway/1 -> ri_to_c/2
  real_gateway/1 -> ri_to_c/1
  c_to_ri/2(im) -> imag_gateway/1  "c_to_ri_out2"
  c_to_ri/1(re) -> real_gateway/1  "c_to_ri_out1"

== system fft_wideband_real/multi_to_workspace_complex/to_workspace_cplx_15 ==
  out15 : Inport
  c_to_ri : Subsystem
  imag_gateway : xbsIndex_r4/Gateway Out  inherit_from_input=on  hdl_port=off  timing_constraint=None  locs_specified=off  LOCs={}  UseAsDAC=off  DACChannel='1'  block_type=gatewayout
  real_gateway : xbsIndex_r4/Gateway Out  inherit_from_input=on  hdl_port=off  timing_constraint=None  locs_specified=off  LOCs={}  UseAsDAC=off  DACChannel='1'  block_type=gatewayout
  ri_to_c : RealImagToComplex
  workspace_output : ToWorkspace  VariableName=out15  SampleTime=-1
  _o : Outport
  wires:
  out15/1 -> c_to_ri/1(c), _o/1
  ri_to_c/1 -> workspace_output/1  "cplx"
  imag_gateway/1 -> ri_to_c/2
  real_gateway/1 -> ri_to_c/1
  c_to_ri/2(im) -> imag_gateway/1  "c_to_ri_out2"
  c_to_ri/1(re) -> real_gateway/1  "c_to_ri_out1"

== system fft_wideband_real/multi_to_workspace_complex/to_workspace_cplx_16 ==
  out16 : Inport
  c_to_ri : Subsystem
  imag_gateway : xbsIndex_r4/Gateway Out  inherit_from_input=on  hdl_port=off  timing_constraint=None  locs_specified=off  LOCs={}  UseAsDAC=off  DACChannel='1'  block_type=gatewayout
  real_gateway : xbsIndex_r4/Gateway Out  inherit_from_input=on  hdl_port=off  timing_constraint=None  locs_specified=off  LOCs={}  UseAsDAC=off  DACChannel='1'  block_type=gatewayout
  ri_to_c : RealImagToComplex
  workspace_output : ToWorkspace  VariableName=out16  SampleTime=-1
  _o : Outport
  wires:
  out16/1 -> c_to_ri/1(c), _o/1
  ri_to_c/1 -> workspace_output/1  "cplx"
  imag_gateway/1 -> ri_to_c/2
  real_gateway/1 -> ri_to_c/1
  c_to_ri/2(im) -> imag_gateway/1  "c_to_ri_out2"
  c_to_ri/1(re) -> real_gateway/1  "c_to_ri_out1"

== system fft_wideband_real/multi_to_workspace_complex/to_workspace_cplx_2 ==
  out2 : Inport
  c_to_ri : Subsystem
  imag_gateway : xbsIndex_r4/Gateway Out  inherit_from_input=on  hdl_port=off  timing_constraint=None  locs_specified=off  LOCs={}  UseAsDAC=off  DACChannel='1'  block_type=gatewayout
  real_gateway : xbsIndex_r4/Gateway Out  inherit_from_input=on  hdl_port=off  timing_constraint=None  locs_specified=off  LOCs={}  UseAsDAC=off  DACChannel='1'  block_type=gatewayout
  ri_to_c : RealImagToComplex
  workspace_output : ToWorkspace  VariableName=out2  SampleTime=-1
  _o : Outport
  wires:
  out2/1 -> c_to_ri/1(c), _o/1
  ri_to_c/1 -> workspace_output/1  "cplx"
  imag_gateway/1 -> ri_to_c/2
  real_gateway/1 -> ri_to_c/1
  c_to_ri/2(im) -> imag_gateway/1  "c_to_ri_out2"
  c_to_ri/1(re) -> real_gateway/1  "c_to_ri_out1"

== system fft_wideband_real/multi_to_workspace_complex/to_workspace_cplx_3 ==
  out3 : Inport
  c_to_ri : Subsystem
  imag_gateway : xbsIndex_r4/Gateway Out  inherit_from_input=on  hdl_port=off  timing_constraint=None  locs_specified=off  LOCs={}  UseAsDAC=off  DACChannel='1'  block_type=gatewayout
  real_gateway : xbsIndex_r4/Gateway Out  inherit_from_input=on  hdl_port=off  timing_constraint=None  locs_specified=off  LOCs={}  UseAsDAC=off  DACChannel='1'  block_type=gatewayout
  ri_to_c : RealImagToComplex
  workspace_output : ToWorkspace  VariableName=out3  SampleTime=-1
  _o : Outport
  wires:
  out3/1 -> c_to_ri/1(c), _o/1
  ri_to_c/1 -> workspace_output/1  "cplx"
  imag_gateway/1 -> ri_to_c/2
  real_gateway/1 -> ri_to_c/1
  c_to_ri/2(im) -> imag_gateway/1  "c_to_ri_out2"
  c_to_ri/1(re) -> real_gateway/1  "c_to_ri_out1"

== system fft_wideband_real/multi_to_workspace_complex/to_workspace_cplx_4 ==
  out4 : Inport
  c_to_ri : Subsystem
  imag_gateway : xbsIndex_r4/Gateway Out  inherit_from_input=on  hdl_port=off  timing_constraint=None  locs_specified=off  LOCs={}  UseAsDAC=off  DACChannel='1'  block_type=gatewayout
  real_gateway : xbsIndex_r4/Gateway Out  inherit_from_input=on  hdl_port=off  timing_constraint=None  locs_specified=off  LOCs={}  UseAsDAC=off  DACChannel='1'  block_type=gatewayout
  ri_to_c : RealImagToComplex
  workspace_output : ToWorkspace  VariableName=out4  SampleTime=-1
  _o : Outport
  wires:
  out4/1 -> c_to_ri/1(c), _o/1
  ri_to_c/1 -> workspace_output/1  "cplx"
  imag_gateway/1 -> ri_to_c/2
  real_gateway/1 -> ri_to_c/1
  c_to_ri/2(im) -> imag_gateway/1  "c_to_ri_out2"
  c_to_ri/1(re) -> real_gateway/1  "c_to_ri_out1"

== system fft_wideband_real/multi_to_workspace_complex/to_workspace_cplx_5 ==
  out5 : Inport
  c_to_ri : Subsystem
  imag_gateway : xbsIndex_r4/Gateway Out  inherit_from_input=on  hdl_port=off  timing_constraint=None  locs_specified=off  LOCs={}  UseAsDAC=off  DACChannel='1'  block_type=gatewayout
  real_gateway : xbsIndex_r4/Gateway Out  inherit_from_input=on  hdl_port=off  timing_constraint=None  locs_specified=off  LOCs={}  UseAsDAC=off  DACChannel='1'  block_type=gatewayout
  ri_to_c : RealImagToComplex
  workspace_output : ToWorkspace  VariableName=out5  SampleTime=-1
  _o : Outport
  wires:
  out5/1 -> c_to_ri/1(c), _o/1
  ri_to_c/1 -> workspace_output/1  "cplx"
  imag_gateway/1 -> ri_to_c/2
  real_gateway/1 -> ri_to_c/1
  c_to_ri/2(im) -> imag_gateway/1  "c_to_ri_out2"
  c_to_ri/1(re) -> real_gateway/1  "c_to_ri_out1"

== system fft_wideband_real/multi_to_workspace_complex/to_workspace_cplx_6 ==
  out6 : Inport
  c_to_ri : Subsystem
  imag_gateway : xbsIndex_r4/Gateway Out  inherit_from_input=on  hdl_port=off  timing_constraint=None  locs_specified=off  LOCs={}  UseAsDAC=off  DACChannel='1'  block_type=gatewayout
  real_gateway : xbsIndex_r4/Gateway Out  inherit_from_input=on  hdl_port=off  timing_constraint=None  locs_specified=off  LOCs={}  UseAsDAC=off  DACChannel='1'  block_type=gatewayout
  ri_to_c : RealImagToComplex
  workspace_output : ToWorkspace  VariableName=out6  SampleTime=-1
  _o : Outport
  wires:
  out6/1 -> c_to_ri/1(c), _o/1
  ri_to_c/1 -> workspace_output/1  "cplx"
  imag_gateway/1 -> ri_to_c/2
  real_gateway/1 -> ri_to_c/1
  c_to_ri/2(im) -> imag_gateway/1  "c_to_ri_out2"
  c_to_ri/1(re) -> real_gateway/1  "c_to_ri_out1"

== system fft_wideband_real/multi_to_workspace_complex/to_workspace_cplx_7 ==
  out7 : Inport
  c_to_ri : Subsystem
  imag_gateway : xbsIndex_r4/Gateway Out  inherit_from_input=on  hdl_port=off  timing_constraint=None  locs_specified=off  LOCs={}  UseAsDAC=off  DACChannel='1'  block_type=gatewayout
  real_gateway : xbsIndex_r4/Gateway Out  inherit_from_input=on  hdl_port=off  timing_constraint=None  locs_specified=off  LOCs={}  UseAsDAC=off  DACChannel='1'  block_type=gatewayout
  ri_to_c : RealImagToComplex
  workspace_output : ToWorkspace  VariableName=out7  SampleTime=-1
  _o : Outport
  wires:
  out7/1 -> c_to_ri/1(c), _o/1
  ri_to_c/1 -> workspace_output/1  "cplx"
  imag_gateway/1 -> ri_to_c/2
  real_gateway/1 -> ri_to_c/1
  c_to_ri/2(im) -> imag_gateway/1  "c_to_ri_out2"
  c_to_ri/1(re) -> real_gateway/1  "c_to_ri_out1"

== system fft_wideband_real/multi_to_workspace_complex/to_workspace_cplx_8 ==
  out8 : Inport
  c_to_ri : Subsystem
  imag_gateway : xbsIndex_r4/Gateway Out  inherit_from_input=on  hdl_port=off  timing_constraint=None  locs_specified=off  LOCs={}  UseAsDAC=off  DACChannel='1'  block_type=gatewayout
  real_gateway : xbsIndex_r4/Gateway Out  inherit_from_input=on  hdl_port=off  timing_constraint=None  locs_specified=off  LOCs={}  UseAsDAC=off  DACChannel='1'  block_type=gatewayout
  ri_to_c : RealImagToComplex
  workspace_output : ToWorkspace  VariableName=out8  SampleTime=-1
  _o : Outport
  wires:
  out8/1 -> c_to_ri/1(c), _o/1
  ri_to_c/1 -> workspace_output/1  "cplx"
  imag_gateway/1 -> ri_to_c/2
  real_gateway/1 -> ri_to_c/1
  c_to_ri/2(im) -> imag_gateway/1  "c_to_ri_out2"
  c_to_ri/1(re) -> real_gateway/1  "c_to_ri_out1"

== system fft_wideband_real/multi_to_workspace_complex/to_workspace_cplx_9 ==
  out9 : Inport
  c_to_ri : Subsystem
  imag_gateway : xbsIndex_r4/Gateway Out  inherit_from_input=on  hdl_port=off  timing_constraint=None  locs_specified=off  LOCs={}  UseAsDAC=off  DACChannel='1'  block_type=gatewayout
  real_gateway : xbsIndex_r4/Gateway Out  inherit_from_input=on  hdl_port=off  timing_constraint=None  locs_specified=off  LOCs={}  UseAsDAC=off  DACChannel='1'  block_type=gatewayout
  ri_to_c : RealImagToComplex
  workspace_output : ToWorkspace  VariableName=out9  SampleTime=-1
  _o : Outport
  wires:
  out9/1 -> c_to_ri/1(c), _o/1
  ri_to_c/1 -> workspace_output/1  "cplx"
  imag_gateway/1 -> ri_to_c/2
  real_gateway/1 -> ri_to_c/1
  c_to_ri/2(im) -> imag_gateway/1  "c_to_ri_out2"
  c_to_ri/1(re) -> real_gateway/1  "c_to_ri_out1"

== system fft_wideband_real/multi_to_workspace_real/to_workspace_1 ==
  adc_data1 : Inport
  gateway : xbsIndex_r4/Gateway Out  inherit_from_input=on  hdl_port=off  timing_constraint=None  locs_specified=off  LOCs={}  UseAsDAC=off  DACChannel='1'  block_type=gatewayout
  workspace_input : ToWorkspace  VariableName=adc_data1  SampleTime=-1
  _o : Outport
  wires:
  adc_data1/1 -> gateway/1, _o/1
  gateway/1 -> workspace_input/1

== system fft_wideband_real/multi_to_workspace_real/to_workspace_10 ==
  adc_data10 : Inport
  gateway : xbsIndex_r4/Gateway Out  inherit_from_input=on  hdl_port=off  timing_constraint=None  locs_specified=off  LOCs={}  UseAsDAC=off  DACChannel='1'  block_type=gatewayout
  workspace_input : ToWorkspace  VariableName=adc_data10  SampleTime=-1
  _o : Outport
  wires:
  adc_data10/1 -> gateway/1, _o/1
  gateway/1 -> workspace_input/1

== system fft_wideband_real/multi_to_workspace_real/to_workspace_11 ==
  adc_data11 : Inport
  gateway : xbsIndex_r4/Gateway Out  inherit_from_input=on  hdl_port=off  timing_constraint=None  locs_specified=off  LOCs={}  UseAsDAC=off  DACChannel='1'  block_type=gatewayout
  workspace_input : ToWorkspace  VariableName=adc_data11  SampleTime=-1
  _o : Outport
  wires:
  adc_data11/1 -> gateway/1, _o/1
  gateway/1 -> workspace_input/1

== system fft_wideband_real/multi_to_workspace_real/to_workspace_12 ==
  adc_data12 : Inport
  gateway : xbsIndex_r4/Gateway Out  inherit_from_input=on  hdl_port=off  timing_constraint=None  locs_specified=off  LOCs={}  UseAsDAC=off  DACChannel='1'  block_type=gatewayout
  workspace_input : ToWorkspace  VariableName=adc_data12  SampleTime=-1
  _o : Outport
  wires:
  adc_data12/1 -> gateway/1, _o/1
  gateway/1 -> workspace_input/1

== system fft_wideband_real/multi_to_workspace_real/to_workspace_13 ==
  adc_data13 : Inport
  gateway : xbsIndex_r4/Gateway Out  inherit_from_input=on  hdl_port=off  timing_constraint=None  locs_specified=off  LOCs={}  UseAsDAC=off  DACChannel='1'  block_type=gatewayout
  workspace_input : ToWorkspace  VariableName=adc_data13  SampleTime=-1
  _o : Outport
  wires:
  adc_data13/1 -> gateway/1, _o/1
  gateway/1 -> workspace_input/1

== system fft_wideband_real/multi_to_workspace_real/to_workspace_14 ==
  adc_data14 : Inport
  gateway : xbsIndex_r4/Gateway Out  inherit_from_input=on  hdl_port=off  timing_constraint=None  locs_specified=off  LOCs={}  UseAsDAC=off  DACChannel='1'  block_type=gatewayout
  workspace_input : ToWorkspace  VariableName=adc_data14  SampleTime=-1
  _o : Outport
  wires:
  adc_data14/1 -> gateway/1, _o/1
  gateway/1 -> workspace_input/1

== system fft_wideband_real/multi_to_workspace_real/to_workspace_15 ==
  adc_data15 : Inport
  gateway : xbsIndex_r4/Gateway Out  inherit_from_input=on  hdl_port=off  timing_constraint=None  locs_specified=off  LOCs={}  UseAsDAC=off  DACChannel='1'  block_type=gatewayout
  workspace_input : ToWorkspace  VariableName=adc_data15  SampleTime=-1
  _o : Outport
  wires:
  adc_data15/1 -> gateway/1, _o/1
  gateway/1 -> workspace_input/1

== system fft_wideband_real/multi_to_workspace_real/to_workspace_16 ==
  adc_data16 : Inport
  gateway : xbsIndex_r4/Gateway Out  inherit_from_input=on  hdl_port=off  timing_constraint=None  locs_specified=off  LOCs={}  UseAsDAC=off  DACChannel='1'  block_type=gatewayout
  workspace_input : ToWorkspace  VariableName=adc_data16  SampleTime=-1
  _o : Outport
  wires:
  adc_data16/1 -> gateway/1, _o/1
  gateway/1 -> workspace_input/1

== system fft_wideband_real/multi_to_workspace_real/to_workspace_2 ==
  adc_data2 : Inport
  gateway : xbsIndex_r4/Gateway Out  inherit_from_input=on  hdl_port=off  timing_constraint=None  locs_specified=off  LOCs={}  UseAsDAC=off  DACChannel='1'  block_type=gatewayout
  workspace_input : ToWorkspace  VariableName=adc_data2  SampleTime=-1
  _o : Outport
  wires:
  adc_data2/1 -> gateway/1, _o/1
  gateway/1 -> workspace_input/1

== system fft_wideband_real/multi_to_workspace_real/to_workspace_3 ==
  adc_data3 : Inport
  gateway : xbsIndex_r4/Gateway Out  inherit_from_input=on  hdl_port=off  timing_constraint=None  locs_specified=off  LOCs={}  UseAsDAC=off  DACChannel='1'  block_type=gatewayout
  workspace_input : ToWorkspace  VariableName=adc_data3  SampleTime=-1
  _o : Outport
  wires:
  adc_data3/1 -> gateway/1, _o/1
  gateway/1 -> workspace_input/1

== system fft_wideband_real/multi_to_workspace_real/to_workspace_4 ==
  adc_data4 : Inport
  gateway : xbsIndex_r4/Gateway Out  inherit_from_input=on  hdl_port=off  timing_constraint=None  locs_specified=off  LOCs={}  UseAsDAC=off  DACChannel='1'  block_type=gatewayout
  workspace_input : ToWorkspace  VariableName=adc_data4  SampleTime=-1
  _o : Outport
  wires:
  adc_data4/1 -> gateway/1, _o/1
  gateway/1 -> workspace_input/1

== system fft_wideband_real/multi_to_workspace_real/to_workspace_5 ==
  adc_data5 : Inport
  gateway : xbsIndex_r4/Gateway Out  inherit_from_input=on  hdl_port=off  timing_constraint=None  locs_specified=off  LOCs={}  UseAsDAC=off  DACChannel='1'  block_type=gatewayout
  workspace_input : ToWorkspace  VariableName=adc_data5  SampleTime=-1
  _o : Outport
  wires:
  adc_data5/1 -> gateway/1, _o/1
  gateway/1 -> workspace_input/1

== system fft_wideband_real/multi_to_workspace_real/to_workspace_6 ==
  adc_data6 : Inport
  gateway : xbsIndex_r4/Gateway Out  inherit_from_input=on  hdl_port=off  timing_constraint=None  locs_specified=off  LOCs={}  UseAsDAC=off  DACChannel='1'  block_type=gatewayout
  workspace_input : ToWorkspace  VariableName=adc_data6  SampleTime=-1
  _o : Outport
  wires:
  adc_data6/1 -> gateway/1, _o/1
  gateway/1 -> workspace_input/1

== system fft_wideband_real/multi_to_workspace_real/to_workspace_7 ==
  adc_data7 : Inport
  gateway : xbsIndex_r4/Gateway Out  inherit_from_input=on  hdl_port=off  timing_constraint=None  locs_specified=off  LOCs={}  UseAsDAC=off  DACChannel='1'  block_type=gatewayout
  workspace_input : ToWorkspace  VariableName=adc_data7  SampleTime=-1
  _o : Outport
  wires:
  adc_data7/1 -> gateway/1, _o/1
  gateway/1 -> workspace_input/1

== system fft_wideband_real/multi_to_workspace_real/to_workspace_8 ==
  adc_data8 : Inport
  gateway : xbsIndex_r4/Gateway Out  inherit_from_input=on  hdl_port=off  timing_constraint=None  locs_specified=off  LOCs={}  UseAsDAC=off  DACChannel='1'  block_type=gatewayout
  workspace_input : ToWorkspace  VariableName=adc_data8  SampleTime=-1
  _o : Outport
  wires:
  adc_data8/1 -> gateway/1, _o/1
  gateway/1 -> workspace_input/1

== system fft_wideband_real/multi_to_workspace_real/to_workspace_9 ==
  adc_data9 : Inport
  gateway : xbsIndex_r4/Gateway Out  inherit_from_input=on  hdl_port=off  timing_constraint=None  locs_specified=off  LOCs={}  UseAsDAC=off  DACChannel='1'  block_type=gatewayout
  workspace_input : ToWorkspace  VariableName=adc_data9  SampleTime=-1
  _o : Outport
  wires:
  adc_data9/1 -> gateway/1, _o/1
  gateway/1 -> workspace_input/1
